simulink model "C705_FLATEARTH_sim"  (R2016a)
settings: Solver=ode23tb  StartTime=0.0  StopTime=t_sim  FixedStep=Ts  RelTol=1e-2
values from neighbouring files (symbols this model uses):
  att0 = [deg2rad(phi0) deg2rad(theta0) deg2rad(psi0)]    [C705_FLATEARTH_init2.m]
  boost = 30000    [C705_CFD_parameter.m]
  C = [-0.00159261761698 -0.0785492193562 0 0 0 0 0 0 -0.0394443854537 -0.0139411758211 0 0 ... (48 elements, 1x48)]    [C705CFDv2.mat]
  C3to4 = [1 -1 1;1 1 1;-1 1 1;-1 -1 1]    [C705_CFD_parameter.m]    (also in C705_FLATEARTH_init2.m)
  C4to3 = (1/4)*[1 1 -1 -1;-1 1 1 -1;1 1 1 1]    [C705_CFD_parameter.m]    (also in C705_FLATEARTH_init2.m)
  d_transisi = 2e3    (= 2000)    [C705_FLATEARTH_init2.m]
  dela_max = deg2rad(10)    [C705_FLATEARTH_init2.m]
  dele_max = deg2rad(10)    [C705_FLATEARTH_init2.m]
  delr_max = deg2rad(10)    [C705_FLATEARTH_init2.m]
  dmdt = -m_fuel/tmax    (= -0.04)    [C705_CFD_parameter.m]
  f_camera = 0.1    [C705_FLATEARTH_init2.m]
  fmax = (10/180)*pi    (= 0.174532925199)    [C705_CFD_parameter.m]    (also in C705_FLATEARTH_init2.m = deg2rad(10))
  k0 = 1    [C705_FLATEARTH_init2.m]
  Khdot = -1    [C705_FLATEARTH_init2.m]
  Ki_ay = -0.0024    [C705_FLATEARTH_init2.m]
  Ki_az = 0.0085    [C705_FLATEARTH_init2.m]
  Ki_psi = 4.1865e-07    [C705_FLATEARTH_init2.m]
  Ki_theta = 2.1878e-7    (= 2.1878e-07)    [C705_FLATEARTH_init2.m]
  Kiphi = 2e-7    (= 2e-07)    [C705_FLATEARTH_init2.m]
  Kp = -1.3248    [C705_FLATEARTH_init2.m]
  Kp_ay = -0.0135    [C705_FLATEARTH_init2.m]
  Kp_az = 0.0119    [C705_FLATEARTH_init2.m]
  Kp_h = 0.45    [C705_FLATEARTH_init2.m]
  Kp_psi = 1.7937    [C705_FLATEARTH_init2.m]
  Kp_theta = 1.7024    [C705_FLATEARTH_init2.m]
  Kphi = 1.8594    [C705_FLATEARTH_init2.m]
  Kq = 3.8200    (= 3.82)    [C705_FLATEARTH_init2.m]
  Kq_theta = -3.1594    [C705_FLATEARTH_init2.m]
  Kr = -10.1447    [C705_FLATEARTH_init2.m]
  Kr_psi = 8.6031    [C705_FLATEARTH_init2.m]
  Lref = 3.675    [C705_CFD_parameter.m]
  m_init = m_full-m_boost    (= 286)    [C705_CFD_parameter.m]
  N = 3    [C705_FLATEARTH_init2.m]
  p0 = [0,0,-h0]    [C705_FLATEARTH_init2.m]
  p1 = [6000,100,-200]    [C705_FLATEARTH_init2.m]
  p2 = [12000,300,-200]    [C705_FLATEARTH_init2.m]
  p3 = [18000,700,-200]    [C705_FLATEARTH_init2.m]
  pt = [24000,1000,0]    [C705_FLATEARTH_init2.m]
  Sref = 0.1711917    [C705_CFD_parameter.m]
  t_activate_del_a = 3    [C705_FLATEARTH_init2.m]
  t_activate_del_e = 5    [C705_FLATEARTH_init2.m]
  t_activate_del_r = 5    [C705_FLATEARTH_init2.m]
  tboost = 3    [C705_FLATEARTH_init2.m]
  TH = 3    [C705_FLATEARTH_init2.m]
  thrust = 910    [C705_CFD_parameter.m]
  Ts_ap = 1/Fs_ap    (= 0.005)    [C705_FLATEARTH_init2.m]
  Ts_guid = 1/Fs_guid    (= 0.005)    [C705_FLATEARTH_init2.m]
  tswitch = 0    [C705_FLATEARTH_init2.m]
  vb0 = [1e-3 0 0]    [C705_FLATEARTH_init2.m]
  wb0 = [0 0 0]    [C705_FLATEARTH_init2.m]
undefined symbols (not defined in the file or in its folder): DiscIntNeverNeededParam, F, GIr, GPr, K1r, K2r, Kda, Ki_h, Ki_p, Kp_p, Light, MIL
libraries: simulink x11, aerolibasang x4, aerolibguid x3, aerolibwind2 x3, aerolibutil x2, aerolibanim x1, aerolibactuator x1, aerolibtransform2 x1, aerolibatmos2 x1, aerolibgravity2 x1, aerolibbdyn x1, aerolibnav x1
(part 2 of 2)

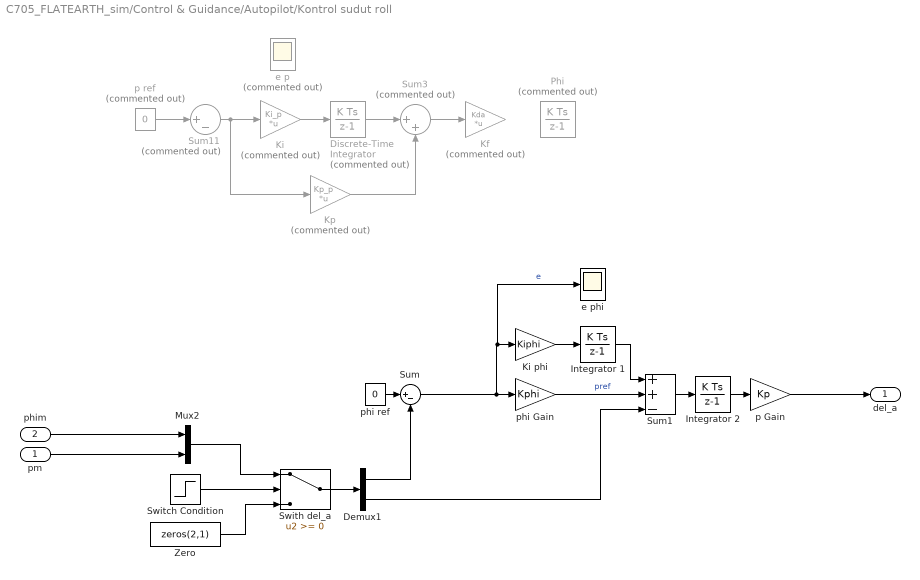
== system C705_FLATEARTH_sim/Control & Guidance/Autopilot/Kontrol sudut roll ==
  pm : Inport
  phim : Inport  Port=2
  "  Integrator 1" : DiscreteIntegrator  InitialConditionSetting=State (most efficient)  SampleTime=Ts_ap  ICPrevOutput=DiscIntNeverNeededParam  ICPrevScaledInput=DiscIntNeverNeededParam
  "  Integrator 2" : DiscreteIntegrator  InitialConditionSetting=State (most efficient)  SampleTime=Ts_ap  ICPrevOutput=DiscIntNeverNeededParam  ICPrevScaledInput=DiscIntNeverNeededParam
  "  Phi" : DiscreteIntegrator  Commented=on  InitialConditionSetting=State (most efficient)  SampleTime=Ts_ap  ICPrevOutput=DiscIntNeverNeededParam  ICPrevScaledInput=DiscIntNeverNeededParam
  Demux1 : Demux  Outputs=2
  Discrete-Time Integrator : DiscreteIntegrator  Commented=on  SampleTime=Ts_ap  ICPrevOutput=DiscIntNeverNeededParam  ICPrevScaledInput=DiscIntNeverNeededParam
  Kf : Gain  Commented=on  Gain=Kda  Multiplication=Matrix(K*u)  SaturateOnIntegerOverflow=on  OutDataTypeStr=Inherit: Same as input  ParamDataTypeStr=Inherit: Same as input
  Ki : Gain  Commented=on  Gain=Ki_p  Multiplication=Matrix(K*u)  SaturateOnIntegerOverflow=on  OutDataTypeStr=Inherit: Same as input  ParamDataTypeStr=Inherit: Same as input
  Ki phi : Gain  Gain=Kiphi
  Kp : Gain  Commented=on  Gain=Kp_p  Multiplication=Matrix(K*u)  SaturateOnIntegerOverflow=on  OutDataTypeStr=Inherit: Same as input  ParamDataTypeStr=Inherit: Same as input
  Mux2 : Mux  Inputs=2
  Sum : Sum  Inputs=|+-  SaturateOnIntegerOverflow=on
  Sum1 : Sum  Inputs=++-  SaturateOnIntegerOverflow=on
  Sum11 : Sum  Commented=on  Inputs=|+-  SaturateOnIntegerOverflow=on  InputSameDT=on  OutDataTypeStr=Inherit: Same as first input
  Sum3 : Sum  Commented=on  Inputs=|++  SaturateOnIntegerOverflow=on  InputSameDT=on  OutDataTypeStr=Inherit: Same as first input
  Switch Condition : Step  Time=t_activate_del_a  Before=-1  SampleTime=0
  Swith del_a : Switch
  Zero : Constant  Value=zeros(2,1)  SampleTime=Ts_guid
  e p : Scope  Commented=on
  e phi : Scope
  p Gain : Gain  Gain=Kp
  p ref : Constant  Commented=on  Value=0
  phi Gain : Gain  Gain=Kphi
  phi ref : Constant  Value=0
  del_a : Outport
  wires:
  Discrete-Time Integrator/1 -> Sum3/1
  Ki/1 -> Discrete-Time Integrator/1
  Sum3/1 -> Kf/1
  Kp/1 -> Sum3/2
  Sum11/1 -> Ki/1, Kp/1
  Sum/1 -> e phi/1, Ki phi/1, phi Gain/1  "e"
  phi Gain/1 -> Sum1/2  "pref"
  p ref/1 -> Sum11/1
  pm/1 -> Mux2/2
  "  Integrator 1"/1 -> Sum1/1
  Ki phi/1 -> "  Integrator 1"/1
  "  Integrator 2"/1 -> p Gain/1
  Sum1/1 -> "  Integrator 2"/1
  phi ref/1 -> Sum/1
  Demux1/1 -> Sum/2
  p Gain/1 -> del_a/1
  Switch Condition/1 -> Swith del_a/2
  Zero/1 -> Swith del_a/3
  Demux1/2 -> Sum1/3
  Swith del_a/1 -> Demux1/1
  Mux2/1 -> Swith del_a/1
  phim/1 -> Mux2/1

== system C705_FLATEARTH_sim/Control & Guidance/Autopilot/Pitch Angle Control ==
  note: Notes:
      | Bila theta diambil dari pengukuran, bukan dari integrasi q,
      | autopilot tidak bekerja dengan baik.
  In : Inport
  Demux1 : Demux  Outputs=2
  Discrete-Time Integrator : DiscreteIntegrator  InitialConditionSetting=State (most efficient)  SampleTime=Ts_ap  ICPrevOutput=DiscIntNeverNeededParam  ICPrevScaledInput=DiscIntNeverNeededParam
  Mux : Mux  Inputs=2
  Sum : Sum  Inputs=|+-  SaturateOnIntegerOverflow=on
  Sum1 : Sum  Inputs=+-  SaturateOnIntegerOverflow=on
  Switch Condition : Step  Time=t_activate_del_e  Before=-1  SampleTime=0
  Switch del_e : Switch
  Theta : DiscreteIntegrator  InitialConditionSetting=State (most efficient)  SampleTime=Ts_ap  ICPrevOutput=DiscIntNeverNeededParam  ICPrevScaledInput=DiscIntNeverNeededParam
  Theta Control : simulink/Continuous/PID Controller  Controller=PI  TimeDomain=Discrete-time  SampleTime=Ts_ap  IntegratorMethod=Trapezoidal  FilterMethod=Forward Euler  Form=Parallel  UseFilter=on  ControllerParametersSource=internal  P=Kp_theta  I=Ki_theta  D=0  N=12  InitialConditionSource=internal  InitialConditionForIntegrator=0  InitialConditionForFilter=0  ExternalReset=none  LimitOutput=off  UpperSaturationLimit=inf  LowerSaturationLimit=-inf  LinearizeAsGain=off  AntiWindupMode=none  Kb=1  TrackingMode=off  Kt=1  PParamMin=[]  PParamMax=[]  IParamMin=[]  IParamMax=[]  DParamMin=[]  DParamMax=[]  NParamMin=[]  NParamMax=[]  KbParamMin=[]  KbParamMax=[]  KtParamMin=[]  KtParamMax=[]  POutMin=[]  POutMax=[]  IOutMin=[]  IOutMax=[]  DOutMin=[]  DOutMax=[]  NOutMin=[]  NOutMax=[]  KbOutMin=[]  KbOutMax=[]  KtOutMin=[]  KtOutMax=[]  IntegratorOutMin=[]  IntegratorOutMax=[]  FilterOutMin=[]  FilterOutMax=[]  SumOutMin=[]  SumOutMax=[]  SumI1OutMin=[]  SumI1OutMax=[]  SumI2OutMin=[]  SumI2OutMax=[]  SumI3OutMin=[]  SumI3OutMax=[]  SumDOutMin=[]  SumDOutMax=[]  SaturationOutMin=[]  SaturationOutMax=[]  IntegratorContinuousStateAttributes=''  IntegratorStateMustResolveToSignalObject=off  IntegratorRTWStateStorageClass=Auto  FilterContinuousStateAttributes=''  FilterStateMustResolveToSignalObject=off  FilterRTWStateStorageClass=Auto  DifferentiatorICPrevScaledInput=0  DifferentiatorOutMin=[]  DifferentiatorOutMax=[]
  Theta Response : Scope
  Zero : Constant  Value=zeros(2,1)  SampleTime=Ts_guid
  "e Theta " : Scope
  q Gain : Gain  Gain=Kq_theta
  del_e : Outport
  wires:
  Theta Control/1 -> Sum1/1
  Sum1/1 -> Discrete-Time Integrator/1
  Sum/1 -> "e Theta "/1, Theta Control/1
  Discrete-Time Integrator/1 -> q Gain/1
  Demux1/1 -> Sum/1, Mux/1  "Theta ref"
  Theta/1 -> Sum/2, Mux/2
  Mux/1 -> Theta Response/1
  q Gain/1 -> del_e/1
  Demux1/2 -> Theta/1, Sum1/2  "q"
  Switch Condition/1 -> Switch del_e/2
  Zero/1 -> Switch del_e/3
  In/1 -> Switch del_e/1
  Switch del_e/1 -> Demux1/1

== system C705_FLATEARTH_sim/Control & Guidance/Autopilot/Yaw Angle Control ==
  In : Inport
  Demux1 : Demux  Outputs=2
  Discrete-Time Integrator : DiscreteIntegrator  InitialConditionSetting=State (most efficient)  SampleTime=Ts_ap  ICPrevOutput=DiscIntNeverNeededParam  ICPrevScaledInput=DiscIntNeverNeededParam
  Mux : Mux  Inputs=2
  Psi : DiscreteIntegrator  InitialConditionSetting=State (most efficient)  SampleTime=Ts_ap  ICPrevOutput=DiscIntNeverNeededParam  ICPrevScaledInput=DiscIntNeverNeededParam
  Psi Control : simulink/Continuous/PID Controller  Controller=PI  TimeDomain=Discrete-time  SampleTime=Ts_ap  IntegratorMethod=Trapezoidal  FilterMethod=Forward Euler  Form=Parallel  UseFilter=on  ControllerParametersSource=internal  P=Kp_psi  I=Ki_psi  D=0  N=12  InitialConditionSource=internal  InitialConditionForIntegrator=0  InitialConditionForFilter=0  ExternalReset=none  LimitOutput=off  UpperSaturationLimit=inf  LowerSaturationLimit=-inf  LinearizeAsGain=off  AntiWindupMode=none  Kb=1  TrackingMode=off  Kt=1  PParamMin=[]  PParamMax=[]  IParamMin=[]  IParamMax=[]  DParamMin=[]  DParamMax=[]  NParamMin=[]  NParamMax=[]  KbParamMin=[]  KbParamMax=[]  KtParamMin=[]  KtParamMax=[]  POutMin=[]  POutMax=[]  IOutMin=[]  IOutMax=[]  DOutMin=[]  DOutMax=[]  NOutMin=[]  NOutMax=[]  KbOutMin=[]  KbOutMax=[]  KtOutMin=[]  KtOutMax=[]  IntegratorOutMin=[]  IntegratorOutMax=[]  FilterOutMin=[]  FilterOutMax=[]  SumOutMin=[]  SumOutMax=[]  SumI1OutMin=[]  SumI1OutMax=[]  SumI2OutMin=[]  SumI2OutMax=[]  SumI3OutMin=[]  SumI3OutMax=[]  SumDOutMin=[]  SumDOutMax=[]  SaturationOutMin=[]  SaturationOutMax=[]  IntegratorContinuousStateAttributes=''  IntegratorStateMustResolveToSignalObject=off  IntegratorRTWStateStorageClass=Auto  FilterContinuousStateAttributes=''  FilterStateMustResolveToSignalObject=off  FilterRTWStateStorageClass=Auto  DifferentiatorICPrevScaledInput=0  DifferentiatorOutMin=[]  DifferentiatorOutMax=[]
  Psi Response : Scope
  Sum : Sum  Inputs=|+-  SaturateOnIntegerOverflow=on
  Sum1 : Sum  Inputs=+-  SaturateOnIntegerOverflow=on
  Switch Condition : Step  Time=t_activate_del_r  Before=-1  SampleTime=0
  Switch del_r : Switch
  Zero : Constant  Value=zeros(2,1)  SampleTime=Ts_guid
  e Psi : Scope
  r Gain : Gain  Gain=Kr_psi
  del_r : Outport
  wires:
  Sum/1 -> e Psi/1, Psi Control/1
  Psi Control/1 -> Sum1/1
  Sum1/1 -> Discrete-Time Integrator/1
  Demux1/1 -> Mux/1, Sum/1  "Psi ref"
  Psi/1 -> Sum/2, Mux/2
  Discrete-Time Integrator/1 -> r Gain/1
  Mux/1 -> Psi Response/1
  Demux1/2 -> Sum1/2, Psi/1  "r"
  r Gain/1 -> del_r/1
  Switch Condition/1 -> Switch del_r/2
  Zero/1 -> Switch del_r/3
  Switch del_r/1 -> Demux1/1
  In/1 -> Switch del_r/1

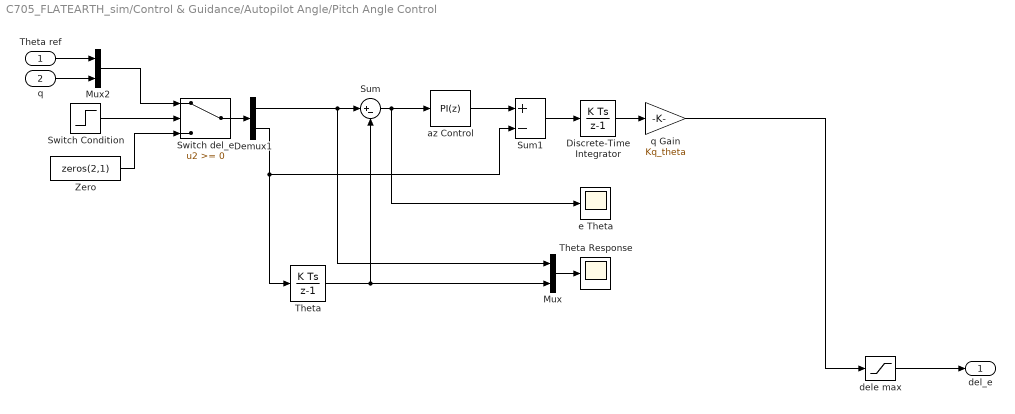
== system C705_FLATEARTH_sim/Control & Guidance/Autopilot Angle/Pitch Angle Control ==
  Theta ref : Inport
  q : Inport  Port=2
  Demux1 : Demux  Outputs=2
  Discrete-Time Integrator : DiscreteIntegrator  InitialConditionSetting=State (most efficient)  SampleTime=Ts_ap  ICPrevOutput=DiscIntNeverNeededParam  ICPrevScaledInput=DiscIntNeverNeededParam
  Mux : Mux  Inputs=2
  Mux2 : Mux  Inputs=2
  Sum : Sum  Inputs=|+-  SaturateOnIntegerOverflow=on
  Sum1 : Sum  Inputs=+-  SaturateOnIntegerOverflow=on
  Switch Condition : Step  Time=t_activate_del_e  Before=-1  SampleTime=0
  Switch del_e : Switch
  Theta : DiscreteIntegrator  InitialConditionSetting=State (most efficient)  SampleTime=Ts_ap  ICPrevOutput=DiscIntNeverNeededParam  ICPrevScaledInput=DiscIntNeverNeededParam
  Theta Response : Scope
  Zero : Constant  Value=zeros(2,1)  SampleTime=Ts_guid
  az Control : simulink/Continuous/PID Controller  Controller=PI  TimeDomain=Discrete-time  SampleTime=Ts_ap  IntegratorMethod=Trapezoidal  FilterMethod=Forward Euler  Form=Parallel  UseFilter=on  ControllerParametersSource=internal  P=Kp_theta  I=Ki_theta  D=0  N=12  InitialConditionSource=internal  InitialConditionForIntegrator=0  InitialConditionForFilter=0  ExternalReset=none  LimitOutput=off  UpperSaturationLimit=inf  LowerSaturationLimit=-inf  LinearizeAsGain=off  AntiWindupMode=none  Kb=1  TrackingMode=off  Kt=1  PParamMin=[]  PParamMax=[]  IParamMin=[]  IParamMax=[]  DParamMin=[]  DParamMax=[]  NParamMin=[]  NParamMax=[]  KbParamMin=[]  KbParamMax=[]  KtParamMin=[]  KtParamMax=[]  POutMin=[]  POutMax=[]  IOutMin=[]  IOutMax=[]  DOutMin=[]  DOutMax=[]  NOutMin=[]  NOutMax=[]  KbOutMin=[]  KbOutMax=[]  KtOutMin=[]  KtOutMax=[]  IntegratorOutMin=[]  IntegratorOutMax=[]  FilterOutMin=[]  FilterOutMax=[]  SumOutMin=[]  SumOutMax=[]  SumI1OutMin=[]  SumI1OutMax=[]  SumI2OutMin=[]  SumI2OutMax=[]  SumI3OutMin=[]  SumI3OutMax=[]  SumDOutMin=[]  SumDOutMax=[]  SaturationOutMin=[]  SaturationOutMax=[]  IntegratorContinuousStateAttributes=''  IntegratorStateMustResolveToSignalObject=off  IntegratorRTWStateStorageClass=Auto  FilterContinuousStateAttributes=''  FilterStateMustResolveToSignalObject=off  FilterRTWStateStorageClass=Auto  DifferentiatorICPrevScaledInput=0  DifferentiatorOutMin=[]  DifferentiatorOutMax=[]
  dele max : Saturate  UpperLimit=dele_max  LowerLimit=-dele_max
  "e Theta " : Scope
  q Gain : Gain  Gain=Kq_theta
  del_e : Outport
  wires:
  az Control/1 -> Sum1/1
  Sum1/1 -> Discrete-Time Integrator/1
  Sum/1 -> "e Theta "/1, az Control/1
  Discrete-Time Integrator/1 -> q Gain/1
  q Gain/1 -> dele max/1
  Demux1/1 -> Sum/1, Mux/1
  Theta/1 -> Sum/2, Mux/2
  Mux/1 -> Theta Response/1
  dele max/1 -> del_e/1
  Demux1/2 -> Theta/1, Sum1/2
  Switch Condition/1 -> Switch del_e/2
  Zero/1 -> Switch del_e/3
  Mux2/1 -> Switch del_e/1
  Switch del_e/1 -> Demux1/1
  Theta ref/1 -> Mux2/1
  q/1 -> Mux2/2

== system C705_FLATEARTH_sim/Control & Guidance/Autopilot Angle/Yaw Angle Control ==
  Psi ref : Inport
  "r " : Inport  Port=2
  Demux1 : Demux  Outputs=2
  Discrete-Time Integrator : DiscreteIntegrator  InitialConditionSetting=State (most efficient)  SampleTime=Ts_ap  ICPrevOutput=DiscIntNeverNeededParam  ICPrevScaledInput=DiscIntNeverNeededParam
  Mux : Mux  Inputs=2
  Mux2 : Mux  Inputs=2
  Psi : DiscreteIntegrator  InitialConditionSetting=State (most efficient)  SampleTime=Ts_ap  ICPrevOutput=DiscIntNeverNeededParam  ICPrevScaledInput=DiscIntNeverNeededParam
  Psi Control : simulink/Continuous/PID Controller  Controller=PI  TimeDomain=Discrete-time  SampleTime=Ts_ap  IntegratorMethod=Trapezoidal  FilterMethod=Forward Euler  Form=Parallel  UseFilter=on  ControllerParametersSource=internal  P=Kp_psi  I=Ki_psi  D=0  N=12  InitialConditionSource=internal  InitialConditionForIntegrator=0  InitialConditionForFilter=0  ExternalReset=none  LimitOutput=off  UpperSaturationLimit=inf  LowerSaturationLimit=-inf  LinearizeAsGain=off  AntiWindupMode=none  Kb=1  TrackingMode=off  Kt=1  PParamMin=[]  PParamMax=[]  IParamMin=[]  IParamMax=[]  DParamMin=[]  DParamMax=[]  NParamMin=[]  NParamMax=[]  KbParamMin=[]  KbParamMax=[]  KtParamMin=[]  KtParamMax=[]  POutMin=[]  POutMax=[]  IOutMin=[]  IOutMax=[]  DOutMin=[]  DOutMax=[]  NOutMin=[]  NOutMax=[]  KbOutMin=[]  KbOutMax=[]  KtOutMin=[]  KtOutMax=[]  IntegratorOutMin=[]  IntegratorOutMax=[]  FilterOutMin=[]  FilterOutMax=[]  SumOutMin=[]  SumOutMax=[]  SumI1OutMin=[]  SumI1OutMax=[]  SumI2OutMin=[]  SumI2OutMax=[]  SumI3OutMin=[]  SumI3OutMax=[]  SumDOutMin=[]  SumDOutMax=[]  SaturationOutMin=[]  SaturationOutMax=[]  IntegratorContinuousStateAttributes=''  IntegratorStateMustResolveToSignalObject=off  IntegratorRTWStateStorageClass=Auto  FilterContinuousStateAttributes=''  FilterStateMustResolveToSignalObject=off  FilterRTWStateStorageClass=Auto  DifferentiatorICPrevScaledInput=0  DifferentiatorOutMin=[]  DifferentiatorOutMax=[]
  Psi Response : Scope
  Sum : Sum  Inputs=|+-  SaturateOnIntegerOverflow=on
  Sum1 : Sum  Inputs=+-  SaturateOnIntegerOverflow=on
  Switch Condition : Step  Time=t_activate_del_r  Before=-1  SampleTime=0
  Switch del_r : Switch
  Zero : Constant  Value=zeros(2,1)  SampleTime=Ts_guid
  delr max : Saturate  UpperLimit=delr_max  LowerLimit=-delr_max
  e Psi : Scope
  r Gain : Gain  Gain=Kr_psi
  del_r : Outport
  wires:
  Sum/1 -> e Psi/1, Psi Control/1
  Psi Control/1 -> Sum1/1
  Sum1/1 -> Discrete-Time Integrator/1
  Demux1/1 -> Mux/1, Sum/1
  Psi/1 -> Sum/2, Mux/2
  Discrete-Time Integrator/1 -> r Gain/1
  r Gain/1 -> delr max/1
  Mux/1 -> Psi Response/1
  Demux1/2 -> Sum1/2, Psi/1
  delr max/1 -> del_r/1
  Switch Condition/1 -> Switch del_r/2
  Zero/1 -> Switch del_r/3
  Mux2/1 -> Switch del_r/1
  Switch del_r/1 -> Demux1/1
  "r "/1 -> Mux2/2
  Psi ref/1 -> Mux2/1

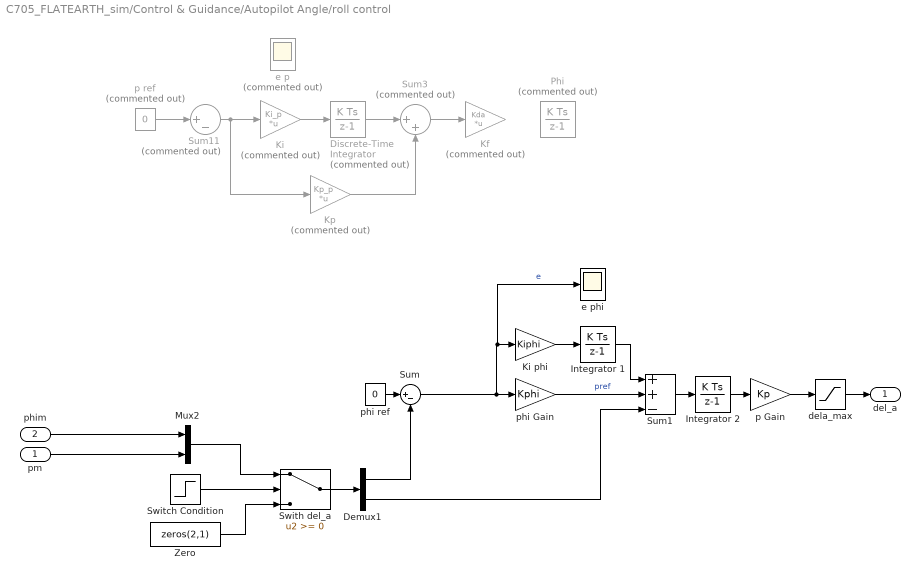
== system C705_FLATEARTH_sim/Control & Guidance/Autopilot Angle/roll control ==
  pm : Inport
  phim : Inport  Port=2
  "  Integrator 1" : DiscreteIntegrator  InitialConditionSetting=State (most efficient)  SampleTime=Ts_ap  ICPrevOutput=DiscIntNeverNeededParam  ICPrevScaledInput=DiscIntNeverNeededParam
  "  Integrator 2" : DiscreteIntegrator  InitialConditionSetting=State (most efficient)  SampleTime=Ts_ap  ICPrevOutput=DiscIntNeverNeededParam  ICPrevScaledInput=DiscIntNeverNeededParam
  "  Phi" : DiscreteIntegrator  Commented=on  InitialConditionSetting=State (most efficient)  SampleTime=Ts_ap  ICPrevOutput=DiscIntNeverNeededParam  ICPrevScaledInput=DiscIntNeverNeededParam
  Demux1 : Demux  Outputs=2
  Discrete-Time Integrator : DiscreteIntegrator  Commented=on  SampleTime=Ts_ap  ICPrevOutput=DiscIntNeverNeededParam  ICPrevScaledInput=DiscIntNeverNeededParam
  Kf : Gain  Commented=on  Gain=Kda  Multiplication=Matrix(K*u)  SaturateOnIntegerOverflow=on  OutDataTypeStr=Inherit: Same as input  ParamDataTypeStr=Inherit: Same as input
  Ki : Gain  Commented=on  Gain=Ki_p  Multiplication=Matrix(K*u)  SaturateOnIntegerOverflow=on  OutDataTypeStr=Inherit: Same as input  ParamDataTypeStr=Inherit: Same as input
  Ki phi : Gain  Gain=Kiphi
  Kp : Gain  Commented=on  Gain=Kp_p  Multiplication=Matrix(K*u)  SaturateOnIntegerOverflow=on  OutDataTypeStr=Inherit: Same as input  ParamDataTypeStr=Inherit: Same as input
  Mux2 : Mux  Inputs=2
  Sum : Sum  Inputs=|+-  SaturateOnIntegerOverflow=on
  Sum1 : Sum  Inputs=++-  SaturateOnIntegerOverflow=on
  Sum11 : Sum  Commented=on  Inputs=|+-  SaturateOnIntegerOverflow=on  InputSameDT=on  OutDataTypeStr=Inherit: Same as first input
  Sum3 : Sum  Commented=on  Inputs=|++  SaturateOnIntegerOverflow=on  InputSameDT=on  OutDataTypeStr=Inherit: Same as first input
  Switch Condition : Step  Time=t_activate_del_a  Before=-1  SampleTime=0
  Swith del_a : Switch
  Zero : Constant  Value=zeros(2,1)  SampleTime=Ts_guid
  dela_max : Saturate  UpperLimit=dela_max  LowerLimit=-dela_max
  e p : Scope  Commented=on
  e phi : Scope
  p Gain : Gain  Gain=Kp
  p ref : Constant  Commented=on  Value=0
  phi Gain : Gain  Gain=Kphi
  phi ref : Constant  Value=0
  del_a : Outport
  wires:
  Discrete-Time Integrator/1 -> Sum3/1
  Ki/1 -> Discrete-Time Integrator/1
  Sum3/1 -> Kf/1
  Kp/1 -> Sum3/2
  Sum11/1 -> Ki/1, Kp/1
  Sum/1 -> e phi/1, Ki phi/1, phi Gain/1  "e"
  phi Gain/1 -> Sum1/2  "pref"
  p ref/1 -> Sum11/1
  pm/1 -> Mux2/2
  "  Integrator 1"/1 -> Sum1/1
  Ki phi/1 -> "  Integrator 1"/1
  "  Integrator 2"/1 -> p Gain/1
  Sum1/1 -> "  Integrator 2"/1
  phi ref/1 -> Sum/1
  Demux1/1 -> Sum/2
  p Gain/1 -> dela_max/1
  Switch Condition/1 -> Swith del_a/2
  Zero/1 -> Swith del_a/3
  Demux1/2 -> Sum1/3
  Swith del_a/1 -> Demux1/1
  Mux2/1 -> Swith del_a/1
  phim/1 -> Mux2/1
  dela_max/1 -> del_a/1

== system C705_FLATEARTH_sim/Custom Variable Mass 6 DOF Flat Earth (Euler)/Calculate DCM & Euler Angles/phidot thetadot psidot  ==
  p q r : Inport
  phi theta psi : Inport  Port=2
  Mux1 : Mux  Inputs=[3 3 3]
  Mux2 : Mux  Inputs=3
  phidot : Fcn  Expr=u[1]+(u[2]*u[4]+u[3]*u[7])*(u[5]/u[8])
  psidot : Fcn  Expr=(u[2]*u[4]+u[3]*u[7])/u[8]
  sincos : Trigonometry  Operator=sincos
  thetadot : Fcn  Expr=u[2]*u[7]-u[3]*u[4]
  phidot thetadot psi : Outport  InitialOutput=0
  wires:
  Mux1/1 -> psidot/1, phidot/1, thetadot/1
  p q r/1 -> Mux1/1
  phi theta psi/1 -> sincos/1
  psidot/1 -> Mux2/3
  thetadot/1 -> Mux2/2
  phidot/1 -> Mux2/1
  Mux2/1 -> phidot thetadot psi/1
  sincos/1 -> Mux1/2
  sincos/2 -> Mux1/3

== system C705_FLATEARTH_sim/Custom Variable Mass 6 DOF Flat Earth (Euler)/Calculate wb_dot /I*wb ==
  p q r : Inport
  Inertia : Inport  Port=2
  Product : Product  Multiplication=Matrix(*)  SaturateOnIntegerOverflow=on  InputSameDT=on  OutDataTypeStr=Inherit: Same as first input
  Reshape1 : Reshape  OutputDimensionality=Column vector (2-D)
  Reshape2 : Reshape
  I * w : Outport
  wires:
  Reshape2/1 -> I * w/1
  Reshape1/1 -> Product/2
  p q r/1 -> Reshape1/1
  Inertia/1 -> Product/1
  Product/1 -> Reshape2/1

== system C705_FLATEARTH_sim/Custom Variable Mass 6 DOF Flat Earth (Euler)/Calculate wb_dot /Idot*wb ==
  I_dot : Inport
  p q r : Inport  Port=2
  Product : Product  Multiplication=Matrix(*)  SaturateOnIntegerOverflow=on  InputSameDT=on  OutDataTypeStr=Inherit: Same as first input
  Reshape1 : Reshape  OutputDimensionality=Column vector (2-D)
  Reshape2 : Reshape
  Id * w : Outport
  wires:
  Reshape2/1 -> Id * w/1
  Reshape1/1 -> Product/2
  Product/1 -> Reshape2/1
  I_dot/1 -> Product/1
  p q r/1 -> Reshape1/1

== matlab function C705_FLATEARTH_sim/Control & Guidance/Camera Seeker/Screen Camera ==
  data: xm input; xs output; att input; xt input; ys output; lamy output; lamz output; f input
% xm missile position in Earth frame
% att missile attitude
% xt target position in Earth frame
% f camera focus length

function [xs,ys,lamy,lamz] = camera(xm,att,xt,f)

a  = xt(1); 
b  = xt(2);
c  = xt(3);

xt2 = [a b c 1]';

phi   = att(1);
theta = att(2);
psi   = att(3);

cx = xm(1);
cy = xm(2);
cz = xm(3);

Cc2w=[cos(theta)*cos(psi)  cos(psi)*sin(phi)*sin(theta)-sin(psi)*cos(phi)  cos(psi)*cos(phi)*sin(theta)+sin(psi)*sin(phi)  0;
      cos(theta)*sin(psi)  sin(psi)*sin(phi)*sin(theta)+cos(psi)*cos(phi)  sin(psi)*cos(phi)*sin(theta)-sin(phi)*cos(psi)  0;  
     -sin(theta)             sin(phi)*cos(theta)                                cos(phi)*cos(theta)  0;
     0                              0                                                    0           1];

 % camera to world
Cw2c=Cc2w';

% camera to image
Tc2i=[1 0 0 0;
      0 f 0 0;
      0 0 f 0];

% translasi  
C=[1 0 0 -cx;
   0 1 0 -cy;
   0 0 1 -cz;
   0 0 0  1];

P = Tc2i*Cw2c*C*xt2; 

% screen coordinate
xs = P(2)/P(1);
ys = -P(3)/P(1);

lamz = atan2(ys,sqrt(xs^2+f^2));
lamy = atan2(xs,f);

end

== matlab function C705_FLATEARTH_sim/Forces and Moments/aerodynamic ==
  data: param input; C input; F output; qbar input; incid input; wb input; del input; M output
function [F,M] = aerodynamic(param,C,qbar,incid,wb,del)

F = zeros(3,1);
M = zeros(3,1);

S = param(1);   % Luasan
L = param(2);   % Panjang

alpha = incid(1)*180/pi;
beta  = incid(2)*180/pi;

del_a = del(1)*180/pi;
del_e = del(2)*180/pi;
del_r = del(3)*180/pi;

p = wb(1);
q = wb(2);
r = wb(3);

% Parameter Aerodinamik
CFX0  = C(1)*alpha+C(2);
CFXda = C(3)*alpha+C(4);
CFXde = C(5)*alpha+C(6);
CFXdr = C(7)*alpha+C(8);

CFY0  = C(9)*beta+C(10);
CFYda = C(11)*alpha+C(12);
CFYde = C(13)*alpha+C(14);
CFYdr = C(15)*alpha+C(16);

CFZ0  = C(17)*alpha+C(18);
CFZda = C(19)*alpha+C(20);
CFZde = C(21)*alpha+C(22);
CFZdr = C(23)*alpha+C(24);

CMX0  = C(25)*beta+C(26);
CMXda = C(27)*alpha+C(28);
CMXde = C(29)*alpha+C(30);
CMXdr = C(31)*alpha+C(32);
CMXp  = C(51);

CMY0  = C(33)*alpha+C(34);
CMYda = C(35)*alpha+C(36);
CMYde = C(37)*alpha+C(38);
CMYdr = C(39)*alpha+C(40);
CMYq  = C(49);

CMZ0  = C(41)*beta+C(42);
CMZda = C(43)*alpha+C(44);
CMZde = C(45)*alpha+C(46);
CMZdr = C(47)*alpha+C(48);
CMZr  = C(50);

CFX = CFX0+CFXda*abs(del_a)+CFXde*del_e     +CFXdr*abs(del_r);
CFY = CFY0+CFYda*abs(del_a)+CFYde*abs(del_e)+CFYdr*del_r;  
CFZ = CFZ0+CFZda*abs(del_a)+CFZde*del_e     +CFZdr*abs(del_r);

CMX = CMX0+CMXda*del_a     +CMXde*abs(del_e)+CMXdr*abs(del_r)+CMXp*p;
CMY = CMY0+CMYda*abs(del_a)+CMYde*del_e     +CMYdr*abs(del_r)+CMYq*q; 
CMZ = CMZ0+CMZda*del_a     +CMZde*abs(del_e)+CMZdr*del_r+CMZr*r; 

FX = qbar*S*CFX;  
FY = qbar*S*CFY;  
FZ = qbar*S*CFZ;  

MX = qbar*S*L*CMX; 
MY = qbar*S*L*CMY; 
MZ = qbar*S*L*CMZ; 

F = [FX FY FZ]';
M = [MX MY MZ]';

end

== matlab function C705_FLATEARTH_sim/Control & Guidance/Guidance ==
  data: aref output; vbm input; wbm input; g input; N input; lamydot input; lamzdot input; dist input; attref output; r input; att input
function [aref,attref] = guidance(vbm,wbm,g,N,lamydot,lamzdot,dist,r,att)

aref   = zeros(3,1);
attref = zeros(3,1);

% Autopilot Percepatan
sigmazdot = lamzdot + wbm(2);
sigmaydot = lamydot + wbm(3);
% sigmaydot = lamydot;
Vm        = norm(vbm);
az        = N*Vm*sigmazdot + g(3);
ay        = N*Vm*sigmaydot + g(2);
aymax     = 50;
azmax     = 50;
if az < 0
    az        = max(az,-azmax);
else
    az        = min(az,azmax);
end
if ay < 0
    ay        = max(ay,-aymax);
else
    ay        = min(ay,aymax);
end
aref    = [0 ay -az]';

% Autopilot Angle
Rx     = dist(1);
Ry     = dist(2);
Rz     = dist(3);
if r > 0
    theta  = asin(-Rz/norm(dist,2))-0; % Tidak digunakan, diganti kontrol ketinggian
    % Angka 0.135 ditentukan dengan trial-error
    % supaya lintasan rudal mendekati jalur waypoint
    psi    = atan2(Ry,Rx);
else
    theta  = lamzdot+att(2); % Tidak digunakan, diganti kontrol ketinggian
    psi    = lamydot+att(3);
end
attref = [0 theta psi]';

end

== matlab function C705_FLATEARTH_sim/Control & Guidance/Virtual Moving Target ==
  data: pos input; vb input; p0 input; p1 input; p2 input; p3 input; p4 input; Ts input; TH input; rw input; k input; rw1 output; k1 output
function [rw1,k1] = waypoint(pos,vb,p0,p1,p2,p3,p4,Ts,TH,rw,k)

if k==1
    r1=p1;
    r2=p2;
elseif k==2
	r1=p2;
    r2=p3;
elseif k==3
	r1=p3;
    r2=p4;
elseif k==4
	r1=p4;
    r2=p4;
else
    r1=p1;
    r2=p2;
end

d=norm(rw-r2);

if (d<10 && k<4)
    k1=k+1;    
else
    k1=k;
end

if k==4
    rw1=p4;
    gm = 0;
    psi = 0;
else
    Rs  = norm(vb)*TH;
    R   = norm(rw-pos);
    V   = norm(vb)*Rs/R;
    
    dx  = r2(1)-r1(1);
    dy  = r2(2)-r1(2);
    dz  = r2(3)-r1(3);
    dxy = sqrt(dy^2+dx^2);
    psi = atan2(dy,abs(dx));
    gm  = atan2(-dz,dxy);
    xw  = rw(1)+V*cos(gm)*cos(psi)*Ts;
    yw  = rw(2)+V*cos(gm)*sin(psi)*Ts;
    zw  = rw(3)-V*sin(gm)*Ts;
    rw1 = [xw yw zw]';
end
